simulink model "EncoderRead_interface"  (R2014b)
settings: Solver=FixedStepDiscrete  StartTime=0.0  StopTime=inf  FixedStep=10^-5  RelTol=1e-3
undefined symbols (not defined in the file): AXI4, Lite
libraries: axiinterfacelib x3
settings Model: FPTRunName=FPA_Reference  SimulationMode=external  Creator=variable  LastModifiedBy=dlwalter
settings SolverCC: PositivePriorityOrder=on
settings DataIOCC: SaveOutput=off  SaveTime=off
settings OptimizationCC: OptimizeModelRefInitCode=on  LifeSpan=1  MaxStackSize=64
settings DebuggingCC: UnderspecifiedInitializationDetection=Classic  MergeDetectMultiDrivingBlocksExec=none
settings HardwareCC: ProdLargestAtomicInteger=Long  ProdLargestAtomicFloat=Double  ProdEndianess=LittleEndian  ProdHWDeviceType=ARM Compatible->ARM Cortex  TargetLargestAtomicInteger=Long  TargetLargestAtomicFloat=Double  TargetIntDivRoundTo=Zero  TargetEndianess=LittleEndian  TargetHWDeviceType=ARMCortex  ProdEqTarget=off
settings RTWCC: SystemTargetFile=ert.tlc  TLCOptions=-aInlineSetEventsForThisBaseRateFcn=TLC_FALSE -aSuppressMultiTaskScheduler=TLC_FALSE  TemplateMakefile=ert_default_tmf  Description=Embedded Coder  ProcessScript=idelink_ert_make_rtw_hook  Toolchain=Xilinx ISE Design Suite 14.4
settings CodeAppCC: IgnoreCustomStorageClasses=off
settings ERTTargetCC: ParMdlRefBuildCompliant=off  GeneratePreprocessorConditionals=Disable all  CPPClassGenCompliant=off  ExtMode=on  ExtModeMexArgs='169.254.1.10'

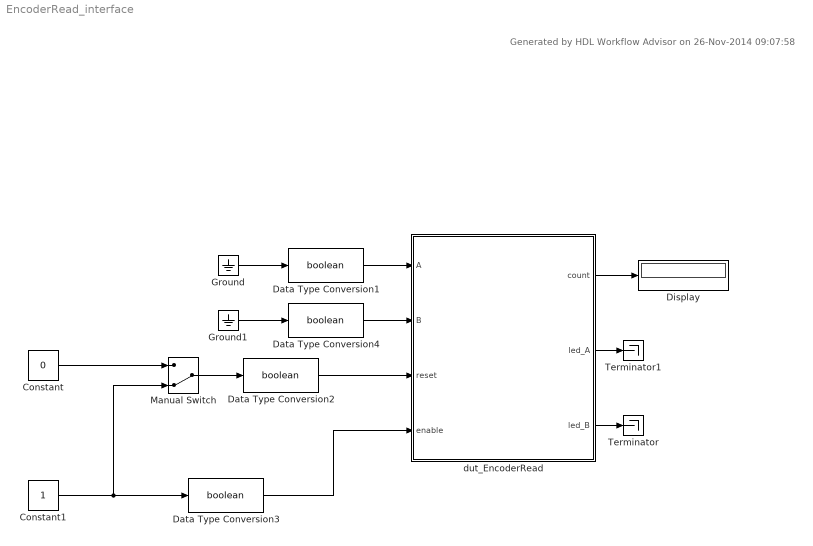
== system EncoderRead_interface ==
  note: Generated by HDL Workflow Advisor on 26-Nov-2014 09:07:58
  Constant : Constant  Value=0  SampleTime=-1
  Constant1 : Constant  SampleTime=-1
  Data Type Conversion{1..4} (4 alike) : DataTypeConversion  OutDataTypeStr=boolean
  Display : Display
  Ground : Ground
  Ground1 : Ground
  Manual Switch : ManualSwitch  CurrentSetting=0
  Terminator : Terminator
  Terminator1 : Terminator
  dut_EncoderRead : Subsystem  TreatAsAtomicUnit=on  MinMaxOverflowLogging=MinMaxAndOverflow  mask(AXI4-Lite/AXI4 Interface){}
      mask help:
      | This is an automatically generated subsystem block.
      | This contains the AXI4-Lite/AXI4 interface which communicates with the encoderread_dut_encoderread_pcore IPCore generated from EncoderRead/dut_EncoderRead subsystem.
      mask Display: disp(sprintf('Xilinx Zynq \nAXI4-Lite/AXI4 Interface'));
  wires:
  Data Type Conversion3/1 -> dut_EncoderRead/4(enable)
  Data Type Conversion2/1 -> dut_EncoderRead/3(reset)
  Ground1/1 -> Data Type Conversion4/1
  Ground/1 -> Data Type Conversion1/1
  Constant1/1 -> Manual Switch/2, Data Type Conversion3/1
  Constant/1 -> Manual Switch/1
  Manual Switch/1 -> Data Type Conversion2/1
  dut_EncoderRead/3(led_B) -> Terminator/1
  dut_EncoderRead/2(led_A) -> Terminator1/1
  dut_EncoderRead/1(count) -> Display/1
  Data Type Conversion1/1 -> dut_EncoderRead/1(A)
  Data Type Conversion4/1 -> dut_EncoderRead/2(B)

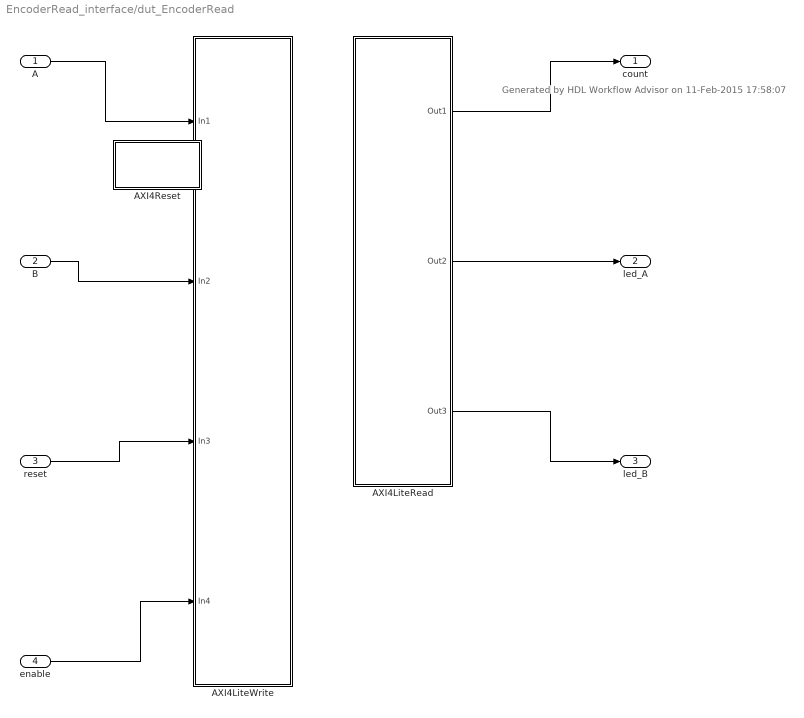
== system EncoderRead_interface/dut_EncoderRead ==
  note: Generated by HDL Workflow Advisor on 11-Feb-2015 17:58:07
  A : Inport
  B : Inport  Port=2
  reset : Inport  Port=3
  enable : Inport  Port=4
  AXI4LiteRead : Subsystem  Priority=10
  AXI4LiteWrite : Subsystem  Priority=1
  AXI4Reset : Subsystem  mask(System Initialize){ShowInLibBrowser=0}
      mask prompts: ShowInLibBrowser "Simulink:masks:CustCodeMaskParam1_MP"
      settings: CopyFcn=cccopyfcn(gcb)  OpenFcn=ccopenfcn('System Initialize Function')
      mask Help: eval('feval(''rtwprivate'',''rtwhelpview'',''rtw_sys_initialize_block'')');
      mask Display: disp('System\nInitialize');
  count : Outport
  led_A : Outport  Port=2
  led_B : Outport  Port=3
  wires:
  A/1 -> AXI4LiteWrite/1(In1)
  B/1 -> AXI4LiteWrite/2(In2)
  reset/1 -> AXI4LiteWrite/3(In3)
  enable/1 -> AXI4LiteWrite/4(In4)
  AXI4LiteRead/1(Out1) -> count/1
  AXI4LiteRead/2(Out2) -> led_A/1
  AXI4LiteRead/3(Out3) -> led_B/1

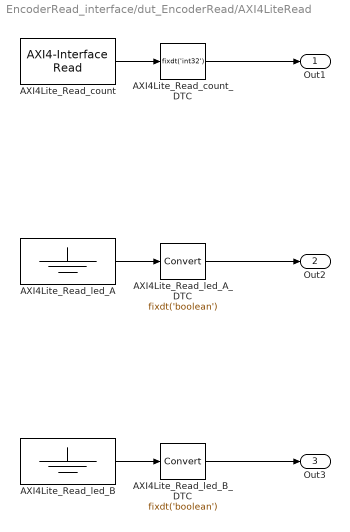
== system EncoderRead_interface/dut_EncoderRead/AXI4LiteRead ==
  AXI4Lite_Read_count : axiinterfacelib/AXI4-Interface Read  Priority=2  AXIInterfaceType=AXI4-Lite  DeviceName=/dev/mwipcore  RegisterOffset=hex2dec('108')  DataType=uint32  DataLength=4096  SampleTime=-1  blockPlatform=ZYNQ  SimulateUsing=Interpreted Execution
  AXI4Lite_Read_count_DTC : DataTypeConversion  OutDataTypeStr=fixdt('int32')  ConvertRealWorld=Stored Integer (SI)
  AXI4Lite_Read_led_A : Ground
  AXI4Lite_Read_led_A_DTC : DataTypeConversion  OutDataTypeStr=fixdt('boolean')  ConvertRealWorld=Stored Integer (SI)
  AXI4Lite_Read_led_B : Ground
  AXI4Lite_Read_led_B_DTC : DataTypeConversion  OutDataTypeStr=fixdt('boolean')  ConvertRealWorld=Stored Integer (SI)
  Out1 : Outport
  Out2 : Outport  Port=2
  Out3 : Outport  Port=3
  wires:
  AXI4Lite_Read_count_DTC/1 -> Out1/1
  AXI4Lite_Read_led_B_DTC/1 -> Out3/1
  AXI4Lite_Read_count/1 -> AXI4Lite_Read_count_DTC/1
  AXI4Lite_Read_led_A/1 -> AXI4Lite_Read_led_A_DTC/1
  AXI4Lite_Read_led_A_DTC/1 -> Out2/1
  AXI4Lite_Read_led_B/1 -> AXI4Lite_Read_led_B_DTC/1

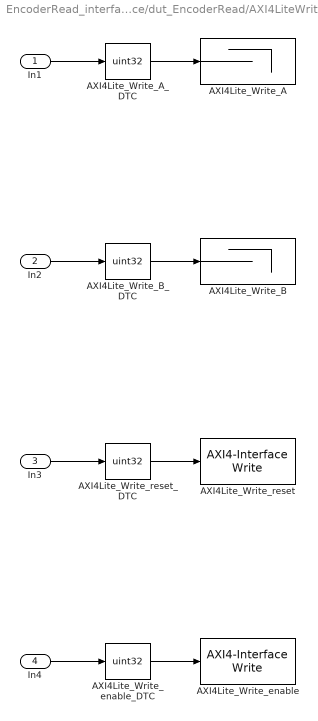
== system EncoderRead_interface/dut_EncoderRead/AXI4LiteWrite ==
  In1 : Inport
  In2 : Inport  Port=2
  In3 : Inport  Port=3
  In4 : Inport  Port=4
  AXI4Lite_Write_A : Terminator
  AXI4Lite_Write_A_DTC : DataTypeConversion  OutDataTypeStr=uint32  ConvertRealWorld=Stored Integer (SI)
  AXI4Lite_Write_B : Terminator
  AXI4Lite_Write_B_DTC : DataTypeConversion  OutDataTypeStr=uint32  ConvertRealWorld=Stored Integer (SI)
  AXI4Lite_Write_enable : axiinterfacelib/AXI4-Interface Write  Priority=4  AXIInterfaceType=AXI4-Lite  DeviceName=/dev/mwipcore  RegisterOffset=hex2dec('104')  blockPlatform=ZYNQ  SimulateUsing=Interpreted execution
  AXI4Lite_Write_enable_DTC : DataTypeConversion  OutDataTypeStr=uint32  ConvertRealWorld=Stored Integer (SI)
  AXI4Lite_Write_reset : axiinterfacelib/AXI4-Interface Write  Priority=3  AXIInterfaceType=AXI4-Lite  DeviceName=/dev/mwipcore  RegisterOffset=hex2dec('100')  blockPlatform=ZYNQ  SimulateUsing=Interpreted execution
  AXI4Lite_Write_reset_DTC : DataTypeConversion  OutDataTypeStr=uint32  ConvertRealWorld=Stored Integer (SI)
  wires:
  AXI4Lite_Write_A_DTC/1 -> AXI4Lite_Write_A/1
  AXI4Lite_Write_reset_DTC/1 -> AXI4Lite_Write_reset/1
  In3/1 -> AXI4Lite_Write_reset_DTC/1
  AXI4Lite_Write_B_DTC/1 -> AXI4Lite_Write_B/1
  In1/1 -> AXI4Lite_Write_A_DTC/1
  In2/1 -> AXI4Lite_Write_B_DTC/1
  In4/1 -> AXI4Lite_Write_enable_DTC/1
  AXI4Lite_Write_enable_DTC/1 -> AXI4Lite_Write_enable/1

== system EncoderRead_interface/dut_EncoderRead/AXI4Reset ==
